simulink model "tp1ej2pE"  (R2024a)
settings: Solver=VariableStepAuto  StartTime=0.0  StopTime=60e-3  MaxStep=5e-6  RelTol=1e-3
undefined symbols (not defined in the file): b, Gs, J, Ka, Kb, Ks, Kt, L, R, Tp, Vref
settings Model: Creator=fab  LastModifiedBy=fab

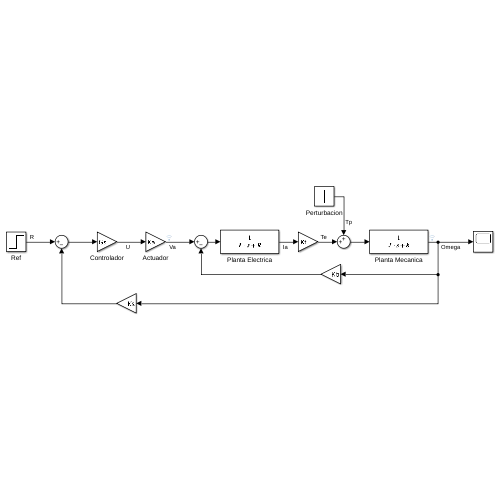
[thumbnail: Simulink's stored preview of the top-level diagram]
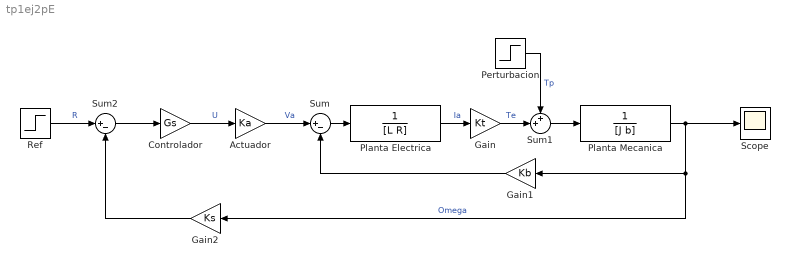
== system tp1ej2pE ==
  Actuador : Gain  Gain=Ka
  Controlador : Gain  Gain=Gs
  Gain : Gain  Gain=Kt
  Gain1 : Gain  Gain=Kb
  Gain2 : Gain  Gain=Ks
  Perturbacion : Step  Time=30e-3  After=Tp  SampleTime=0
  Planta Electrica : TransferFcn  Denominator=[L R]
  Planta Mecanica : TransferFcn  Denominator=[J b]
  Ref : Step  Time=0  After=Vref  SampleTime=0
  Scope : Scope
  Sum : Sum  Inputs=|+-
  Sum1 : Sum  Inputs=++|
  Sum2 : Sum  Inputs=|+-
  wires:
  Controlador/1 -> Actuador/1  "U"
  Ref/1 -> Sum2/1  "R"
  Actuador/1 -> Sum/1  "Va"
  Gain1/1 -> Sum/2
  Gain/1 -> Sum1/2  "Te"
  Sum/1 -> Planta Electrica/1
  Planta Mecanica/1 -> Scope/1, Gain2/1, Gain1/1  "Omega"
  Planta Electrica/1 -> Gain/1  "Ia"
  Sum1/1 -> Planta Mecanica/1
  Perturbacion/1 -> Sum1/1  "Tp"
  Gain2/1 -> Sum2/2
  Sum2/1 -> Controlador/1
